simulink model "Feuchtesimulation_G21_EU6AGA_rueckgabewerte"  (R2021b)
settings: Solver=FixedStepAuto  StartTime=start_time  StopTime=stop_time  FixedStep=ts  RelTol=1e-3
undefined symbols (not defined in the file or in its folder): A_Kat0, A_Kat1, A_Kat2, A_Kat3, A_Mantel_Kat0, A_Mantel_Kat1, A_Mantel_Kat2, A_Mantel_Kat3, Air_N2, Air_O2, beladungskennfeld, C_mw, CO2_mw, FeuchteAnsaugluft_rel, FeuchtegradAnsaugluft, Fuel_C, Fuel_H, H2O_mw, H_mw, Kat0_Anzahl_Zonen, Kat1_Anzahl_Zonen, Kat2_Anzahl_Zonen, Kat3_Anzahl_Zonen, l_Kat0, l_Kat1, l_Kat2, l_Kat3, m_Canning_Kat0, m_Canning_Kat1, m_Canning_Kat2, m_Canning_Kat3, m_h2o_kat0_ads, m_h2o_kat0_kond, m_h2o_kat1_ads, m_h2o_kat1_kond, m_h2o_kat2_ads, m_h2o_kat2_kond, m_h2o_kat3_ads, m_h2o_kat3_kond, m_Isolierung_Kat0, m_Isolierung_Kat1, m_Isolierung_Kat2, m_Isolierung_Kat3, m_zeolith_kat0_zone, m_zeolith_kat1_zone, m_zeolith_kat2_zone, m_zeolith_kat3_zone, m_zKat0, m_zKat1, m_zKat2, m_zKat3, Mat_Kat0, Mat_Kat1, Mat_Kat2, Mat_Kat3, N2_mw, O2_mw, p_dsat, Rohr0, Rohr1 ... (+20)
libraries: Feuchtesimulation_Lib x69
(part 1 of 3)
settings Model: SimulationMode=rapid-accelerator  NumberOfSteps=2  SnapshotInterval=1  Creator=QXS2633  LastModifiedBy=q552088
settings SolverCC: AlgebraicLoopSolver=TrustRegion
settings DataIOCC: Decimation=ScopeDecim  SaveOutput=off  SignalLogging=off  DSMLogging=off  SaveTime=off  ReturnWorkspaceOutputs=off
settings DebuggingCC: SFMachineParentedDataDiag=warning  ArithmeticOperatorsInVariantConditions=warning
settings SFSimCC: CustomCodeUndefinedFunction=UseInterfaceOnly

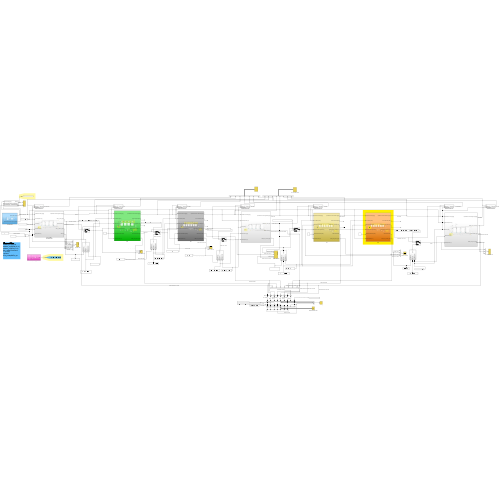
[thumbnail: Simulink's stored preview of the top-level diagram]
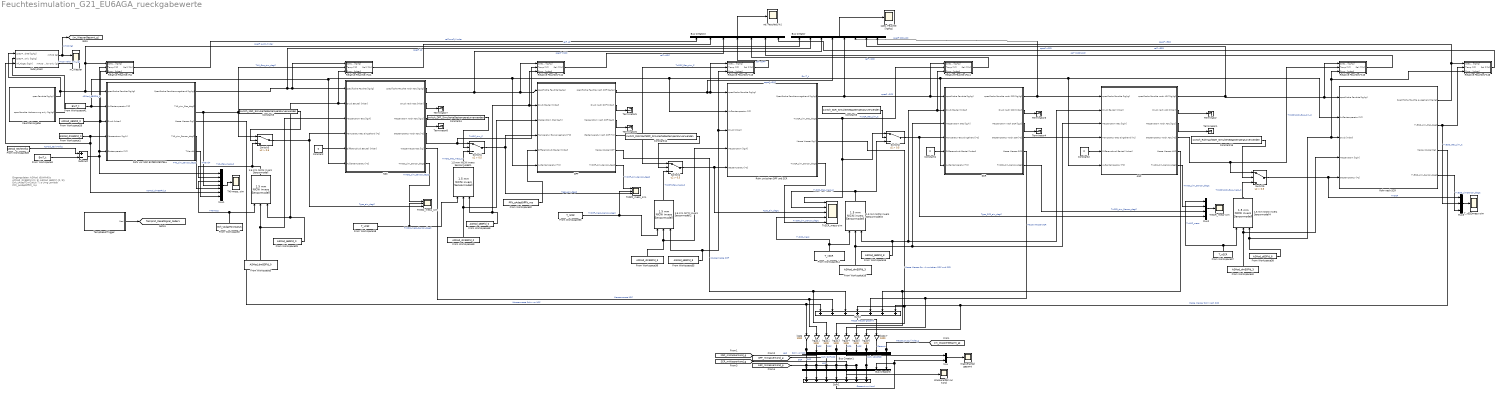
== system Feuchtesimulation_G21_EU6AGA_rueckgabewerte ==
  note: Eingangsdaten:
      | ASMod_tExhMnfUs
      | ASMod_dmEGFld {0 / 3}
      | ASMod_pEGFld {0 / 8}
      | Exh_tAdapTOxiCatUs
      | T / p Umg
      | Lambda
      | PFlt_pAdapDiffFlt_mp
  1.5 mm NiCNi invers Sensormodell{,1..4} (5 alike) : Feuchtesimulation_Lib/1.5 mm NiCNi invers Sensormodell  SystemSampleTime=-1  VariantActivationTime=update diagram  Latency=0  AutoFrameSizeCalculation=off
  ASC : Subsystem
  Bus Creator : BusCreator  Inputs=8
  Bus Creator1 : BusCreator  Inputs=9
  Bus Creator2 : BusCreator  Inputs=7
  Bus Creator3 : BusCreator  Inputs=9
  Constant : Constant  Value=0
  Constant1 : Constant  Value=0
  Constant14 : Constant  Value=switch_RohrNachDPF_SimulierteGastemperaturverwenden
  Constant15 : Constant  Value=switch_RohrnachSCR_SimulierteGastemperaturverwenden
  Constant2 : Constant  Value=0
  Constant3 : Constant  Value=switch_NSC_SimulierteGastemperaturverwenden
  Constant4 : Constant  Value=switch_DPF_SimulierteGastemperaturverwenden
  Constant5 : Constant  Value=switch_SCR_SimulierteGastemperaturverwenden
  DPF : Subsystem
  FeuchteVorgabe : Subsystem
  From Workspace1 : FromWorkspace  VariableName=ASMod_dmEGFld_0  OutputAfterFinalValue=Holding final value
  From Workspace14 : FromWorkspace  VariableName=T_vSCR  OutputAfterFinalValue=Holding final value
  From Workspace15 : FromWorkspace  VariableName=ASMod_pEGFld_8  OutputAfterFinalValue=Holding final value
  From Workspace16 : FromWorkspace  VariableName=ASMod_dmEGFld_3  OutputAfterFinalValue=Holding final value
  From Workspace18 : FromWorkspace  VariableName=T_vCSF  OutputAfterFinalValue=Holding final value
  From Workspace2 : FromWorkspace  VariableName=Exh_tAdapTOxiCatUs  OutputAfterFinalValue=Holding final value
  From Workspace26 : FromWorkspace  VariableName=ASMod_pEGFld_0  OutputAfterFinalValue=Holding final value
  From Workspace28 : FromWorkspace  VariableName=ASMod_tExhMnfUs  OutputAfterFinalValue=Holding final value
  From Workspace29 : FromWorkspace  VariableName=ASMod_pEGFld_0  OutputAfterFinalValue=Holding final value
  From Workspace3 : FromWorkspace  VariableName=EnvT_t
  From Workspace32 : FromWorkspace  VariableName=PFlt_pAdapDiffFlt_mp  OutputAfterFinalValue=Holding final value
  From Workspace33 : FromWorkspace  VariableName=T_nCSF  OutputAfterFinalValue=Holding final value
  From Workspace35 : FromWorkspace  VariableName=ASMod_pEGFld_8  OutputAfterFinalValue=Holding final value
  From Workspace36 : FromWorkspace  VariableName=ASMod_dmEGFld_3  OutputAfterFinalValue=Holding final value
  From Workspace37 : FromWorkspace  VariableName=T_nSCR  OutputAfterFinalValue=Holding final value
  From Workspace38 : FromWorkspace  VariableName=ASMod_pEGFld_8  OutputAfterFinalValue=Holding final value
  From Workspace40 : FromWorkspace  VariableName=ASMod_dmEGFld_3  OutputAfterFinalValue=Holding final value
  From Workspace41 : FromWorkspace  VariableName=EnvT_t  OutputAfterFinalValue=Holding final value
  From Workspace48 : FromWorkspace  VariableName=ASMod_pEGFld_0  OutputAfterFinalValue=Holding final value
  From Workspace49 : FromWorkspace  VariableName=ASMod_dmEGFld_0  OutputAfterFinalValue=Holding final value
  From Workspace5 : FromWorkspace  VariableName=ASMod_dmEGFld_0  OutputAfterFinalValue=Holding final value
  Mux : Mux  Inputs=2
  Mux1 : Mux  Inputs=7
  Mux2 : Mux
  Mux3 : Mux  Inputs=3
  NSC : Subsystem
  Relative Feuchte [%] : Subsystem
  Relative Feuchte [%]1 : Subsystem
  Relative Feuchte [%]2 : Subsystem
  Relative Feuchte [%]3 : Subsystem
  Relative Feuchte [%]4 : Subsystem
  Relative Feuchte [%]5 : Subsystem
  Relative Feuchte [%]6 : Subsystem
  Rohr nach SCR : Subsystem
  Rohr vor NSC EXPERIMENTELL : Subsystem
  Rohr zwischen DPF und SCR : Subsystem
  SCR : Subsystem
  Subsystem : Subsystem
  Subtract : Sum  Inputs=+-
  Sum1 : Sum  Inputs=+++++++
  Sum2 : Sum  Inputs=+++++++
  Switch{1..5} (5 alike) : Switch  Criteria=u2 > Threshold  Threshold=0.5  RndMeth=Simplest  SaturateOnIntegerOverflow=on  InputSameDT=on
  "T40 mess, sim" : Scope
  T_vESDmess-sim : Scope
  TempResetTrigger : Subsystem
  Terminator{,1,3..8} (8 alike) : Terminator
  TnDPF_mess_sim : Scope  NumInputPorts=3
  TnNSC_mess_sim : Scope  NumInputPorts=3
  TnSCR_mess-sim : Scope
  TvSCR_mess-sim : Scope  NumInputPorts=5
  Wasseranfall gesamt : Scope
  Wasseranfall nur Kond : Scope
  kg2g {,1..7} (8 alike) : Gain  Gain=1000
  m_Wasser : Scope  NumInputPorts=2
  rel. Feuchte [%] : Scope
  spez. Feuchte [kg/kg] : Scope
  tag scope: TempInit_ResetSignal_0oder1=global
  wires:
  Sum2/1 -> kg2g 7/1  "Masse Wasser gesamt"
  NSC/3(Massenstrom nach NSC [kg/s]) -> Terminator8/1
  [SCR_mWasserKond_g] -> Sum1/5, Bus Creator3/5  "SCR"
  Constant2/1 -> ASC/5(Differenzdruck Bauteil [mbar])
  Bus Creator3/1 -> Wasseranfall nur Kond/1
  Relative Feuchte [%]2/1(Rel F [%]) -> Bus Creator2/3  "relF nNSC"
  Sum1/1 -> Mux/2, Bus Creator3/8  "Gesamt nur Kond"
  kg2g 4/1 -> Bus Creator1/5  "SCR"
  Constant5/1 -> Switch2/2
  Rohr zwischen DPF und SCR/3(Masse Wasser [kg]) -> kg2g 3/1, Sum2/4  "Masse Wasser Rorh zwischen DPF und SCR"
  SCR/1(spezifische Feuchte nach SCR [kg/kg]) -> ASC/1(spezifische Feuchte [kg/kg]), Bus Creator/6  "spezF SCR-ASC"
  Rohr nach SCR/3(Masse Wasser [kg]) -> Sum2/7, kg2g 6/1  "Masse Wasser Rohr nach SCR"
  Switch5/1 -> Rohr nach SCR/5(Gastemperatur [°C]), Mux3/1  "TnSCR"
  [m_WasserGesamt_g] -> Bus Creator3/9, Bus Creator1/9  "Wasser_ausZylinder_g"
  ASC/3(Massenstrom nach ASC [kg/s]) -> Terminator1/1
  SCR/2(Druck nach SCR [mbar]) -> Terminator3/1
  ASC/2(Druck nach ASC [mbar]) -> Terminator/1
  kg2g 3/1 -> Sum1/4, Bus Creator3/4, Bus Creator1/4  "Rohr DPF-SCR"
  Relative Feuchte [%]4/1(Rel F [%]) -> Bus Creator2/5  "relF vSCR"
  [NSC_mWasserKond_g] -> Sum1/2, Bus Creator3/2  "NSC"
  Subsystem/1(mH2O [g]) -> m_Wasser/1, [m_WasserGesamt_g]  "mH2O [g]"
  kg2g 6/1 -> Sum1/7, Bus Creator3/7, Bus Creator1/7  "Rohr ASC-ESD"
  "kg2g "/1 -> Sum1/1, Bus Creator3/1, Bus Creator1/1  "Rohr vor NSC"
  Relative Feuchte [%]/1(Rel F [%]) -> Bus Creator2/1  "relF ausZylinder"
  Bus Creator1/1 -> Mux/1
  SCR/3(Massenstrom nach SCR [kg/s]) -> Terminator4/1
  Relative Feuchte [%]3/1(Rel F [%]) -> Bus Creator2/4  "relF nDPF"
  FeuchteVorgabe/2(spez.Feuchte Verbrennung only [kg/kg]) -> Subsystem/2(spez-Feuchte Verbrennung only [kg/kg])
  DPF/3(Massenstrom nach DPF [kg/s]) -> Terminator6/1
  Rohr nach SCR/1(Spezifische Feuchte ausgehend [kg/kg]) -> Relative Feuchte [%]6/1(Spez F [kg/kg]), Bus Creator/8  "spezF vESD"
  DPF/4(Gastemperatur nach DPF [°C]) -> Switch4/1, Relative Feuchte [%]3/2(Temp [°C])  "TnDPF_Gas_sim_C"
  Constant15/1 -> Switch5/2
  [DPF_mWasserKond_g] -> Sum1/3, Bus Creator3/3  "DPF"
  kg2g 5/1 -> Bus Creator1/6  "ASC"
  ASC/4(Gastemperatur nach ASC [°C]) -> Relative Feuchte [%]5/2(Temp [°C]), Switch5/1  "TnSCR(ASC)_Gas_sim_C"
  FeuchteVorgabe/1(spez.Feuchte [kg/kg]) -> Subsystem/1(spez-Feuchte [kg/kg]), Bus Creator/1, Relative Feuchte [%]/1(Spez F [kg/kg]), Rohr vor NSC EXPERIMENTELL/1(spezifische Feuchte [kg/kg])  "spezF ausZylinder"
  Switch3/1 -> TnNSC_mess_sim/3, NSC/4(Temperatur Gas eingehend [°C])  "Tgas_ein_degC"
  ASC/5(Masse Wasser ASC) -> Sum2/6, kg2g 5/1
  kg2g 7/1 -> Bus Creator1/8  "Gesamt"
  From Workspace18/1 -> TnNSC_mess_sim/2, 1.5 mm NiCNi invers Sensormodell1/1  "TnNSC_mess_Sensor_degC"
  Rohr vor NSC EXPERIMENTELL/2(T40_sim_Gas_degC) -> Mux1/4, Switch3/1, Relative Feuchte [%]1/2(Temp [°C])  "T40_Gas_sim_degC"
  1.5 mm NiCNi invers Sensormodell2/1 -> Switch4/3  "TnDPF_Gas_mess_C"
  1.5 mm NiCNi invers Sensormodell4/1 -> Switch5/3  "TnSCR(ASC)_Gas_mess_C"
  Switch4/1 -> TvSCR_mess-sim/3, Rohr zwischen DPF und SCR/5(Gastemperatur [°C])  "Tgas_ein_degC"
  Rohr zwischen DPF und SCR/2(TvSCR_sim_Gas_degC) -> Relative Feuchte [%]4/2(Temp [°C]), TvSCR_mess-sim/1, Switch2/1  "TvSCR_Gas_sim_C"
  NSC/2(Druck nach NSC [mbar]) -> Terminator7/1
  Relative Feuchte [%]5/1(Rel F [%]) -> Bus Creator2/6  "relF nSCR(ASC)"
  Rohr nach SCR/2(TvESD_sim_Gas_degC) -> Relative Feuchte [%]6/2(Temp [°C]), Mux3/2  "TvESD_Gas_sim_C"
  DPF/2(Druck nach DPF [mbar]) -> Terminator5/1
  Rohr vor NSC EXPERIMENTELL/3(Masse Wasser [kg]) -> "kg2g "/1, Sum2/1  "Wassermasse Rohr vor NSC"
  Rohr vor NSC EXPERIMENTELL/1(Spezifische Feuchte ausgehend [kg/kg]) -> Bus Creator/2, Relative Feuchte [%]1/1(Spez F [kg/kg]), NSC/1(spezifische Feuchte [kg/kg])  "spezF 40"
  Switch2/1 -> Mux2/4, SCR/4(Temperatur Gas eingehend [°C])  "Tgas_SCR_ein_degC"
  [ASC_mWasserKond_g] -> Sum1/6, Bus Creator3/6  "ASC"
  From Workspace41/1 -> NSC/6(Außentemperatur [°C]), SCR/6(Außentemperatur [°C]), Rohr nach SCR/2(Außentemperatur [°C]), ASC/6(Außentemperatur [°C]), Rohr zwischen DPF und SCR/2(Außentemperatur [°C]), DPF/6(Außentemperatur [°C]), Rohr vor NSC EXPERIMENTELL/2(Außentemperatur [°C])  "EnvT_t"
  From Workspace28/1 -> Subtract/1  "ASMod_tExhMnfUs"
  Rohr zwischen DPF und SCR/1(Spezifische Feuchte ausgehend [kg/kg]) -> Relative Feuchte [%]4/1(Spez F [kg/kg]), SCR/1(spezifische Feuchte [kg/kg]), Bus Creator/5  "spezF vSCR"
  Bus Creator2/1 -> rel. Feuchte [%]/1
  From Workspace1/1 -> Mux1/6, Subsystem/3(mf_Abgas [kg/h]), Rohr vor NSC EXPERIMENTELL/4(Massenstrom [kg/h])  "ASMod_dmEGFld_0"
  From Workspace37/1 -> Mux2/1, 1.5 mm NiCNi invers Sensormodell4/1  "TnASC_mess"
  From Workspace26/1 -> Relative Feuchte [%]/3(Druck [mbar]), Rohr vor NSC EXPERIMENTELL/3(Druck [mbar])  "ASMod_pEGFld_0"
  From Workspace29/1 -> Relative Feuchte [%]1/3(Druck [mbar]), NSC/2(Druck Bauteil [mbar]), 1.5 mm NiCNi invers Sensormodell/3
  Subsystem/2(mH2O Verbr.-only [g]) -> m_Wasser/2  "mH2O Verbr. only [g]"
  Mux/1 -> Wasseranfall gesamt/1
  ASC/1(spezifische Feuchte nach ASC [kg/kg]) -> Relative Feuchte [%]5/1(Spez F [kg/kg]), Rohr nach SCR/1(spezifische Feuchte [kg/kg]), Bus Creator/7  "spezF nSCR"
  From Workspace33/1 -> TnDPF_mess_sim/2, 1.5 mm NiCNi invers Sensormodell2/1  "TnDPF_mess_Sensor_degC"
  DPF/1(spezifische Feuchte nach DPF [kg/kg]) -> Rohr zwischen DPF und SCR/1(spezifische Feuchte [kg/kg]), Relative Feuchte [%]3/1(Spez F [kg/kg]), Bus Creator/4  "spezF nDPF"
  Relative Feuchte [%]1/1(Rel F [%]) -> Bus Creator2/2  "relF 40"
  NSC/1(spezifische Feuchte nach NSC [kg/kg]) -> Bus Creator/3, Relative Feuchte [%]2/1(Spez F [kg/kg]), DPF/1(spezifische Feuchte [kg/kg])  "spezF nNSC"
  DPF/5(Masse Wasser DPF) -> kg2g 2/1, Sum2/3  "Wassermasse DPF"
  From Workspace38/1 -> Relative Feuchte [%]6/3(Druck [mbar]), Relative Feuchte [%]5/3(Druck [mbar]), Rohr nach SCR/3(Druck [mbar]), 1.5 mm NiCNi invers Sensormodell4/3
  From Workspace2/1 -> Mux1/3, 1.5 mm NiCNi invers Sensormodell/1  "T40mess"
  1.5 mm NiCNi invers Sensormodell/1 -> Mux1/2, Switch3/3  "T40_Gas_mess_C"
  NSC/5(Wassermasse NSC [kg]) -> kg2g 1/1, Sum2/2  "Wassermasse NSC"
  Constant4/1 -> Switch1/2
  kg2g 2/1 -> Bus Creator1/3  "DPF"
  Constant3/1 -> Switch3/2
  From Workspace15/1 -> ASC/2(Druck Bauteil [mbar]), Relative Feuchte [%]4/3(Druck [mbar]), SCR/2(Druck Bauteil [mbar]), 1.5 mm NiCNi invers Sensormodell3/3
  From Workspace40/1 -> Rohr nach SCR/4(Massenstrom [kg/h]), 1.5 mm NiCNi invers Sensormodell4/2
  NSC/6(TnNSC_sim_Sensor_degC) -> TnNSC_mess_sim/1  "TnNSC_sim_Sensor_degC"
  Constant14/1 -> Switch4/2
  From Workspace36/1 -> Rohr zwischen DPF und SCR/4(Massenstrom [kg/h]), 1.5 mm NiCNi invers Sensormodell2/2
  From Workspace48/1 -> DPF/2(Druck Bauteil [mbar]), Relative Feuchte [%]2/3(Druck [mbar]), 1.5 mm NiCNi invers Sensormodell1/3
  From Workspace35/1 -> Relative Feuchte [%]3/3(Druck [mbar]), Rohr zwischen DPF und SCR/3(Druck [mbar]), 1.5 mm NiCNi invers Sensormodell2/3
  1.5 mm NiCNi invers Sensormodell1/1 -> Switch1/3  "TnNSC_Gas_mess_C"
  Bus Creator/1 -> spez. Feuchte [kg/kg]/1
  NSC/4(Gastemperatur nach NSC [°C]) -> Relative Feuchte [%]2/2(Temp [°C]), Switch1/1  "TnNSC_sim_C"
  From Workspace32/1 -> DPF/5(Differenzdruck Bauteil [mbar])
  SCR/4(Gastemperatur nach SCR [°C]) -> ASC/4(Temperatur Gas eingehend [°C])
  kg2g 1/1 -> Bus Creator1/2  "NSC"
  From Workspace49/1 -> DPF/3(Massenstrom Gas [kg/h]), 1.5 mm NiCNi invers Sensormodell1/2
  From Workspace14/1 -> TvSCR_mess-sim/4, 1.5 mm NiCNi invers Sensormodell3/1  "TvSCR_mess"
  1.5 mm NiCNi invers Sensormodell3/1 -> TvSCR_mess-sim/2, Switch2/3  "TvSCR_Gas_mess_C"
  SCR/5(Masse Wasser SCR) -> Sum2/5, kg2g 4/1  "Masse Wasser SCR"
  Switch1/1 -> TnDPF_mess_sim/3, DPF/4(Temperatur Gas eingehend [°C])  "Tgas_ein_degC"
  ASC/6(TnASC_sim_Sensor_degC) -> Mux2/2  "TnASC_sim_Sensor_degC"
  Constant1/1 -> SCR/5(Differenzdruck Bauteil [mbar])
  From Workspace16/1 -> ASC/3(Massenstrom Gas [kg/h]), SCR/3(Massenstrom Gas [kg/h]), 1.5 mm NiCNi invers Sensormodell3/2
  Constant/1 -> NSC/5(Differenzdruck Bauteil [mbar])
  From Workspace5/1 -> NSC/3(Massenstrom Gas [kg/h]), 1.5 mm NiCNi invers Sensormodell/2
  TempResetTrigger/1(Resi) -> [TempInit_ResetSignal_0oder1]
  Mux1/1 -> "T40 mess, sim"/1
  Rohr vor NSC EXPERIMENTELL/4(T40_sim_Sensor_degC) -> Mux1/5  "T40_sim_Sensor_degC"
  DPF/6(TnDPF_sim_Sensor_degC) -> TnDPF_mess_sim/1  "TnDPF_sim_Sensor_degC"
  Rohr zwischen DPF und SCR/4(TvSCR_sim_Sensor_degC) -> TvSCR_mess-sim/5  "TvSCR_sim_Sensor_degC"
  Mux2/1 -> TnSCR_mess-sim/1
  SCR/6(TnSCR_sim_Sensor_degC) -> Mux2/3  "TnSCR_sim_Sensor_degC"
  Mux3/1 -> T_vESDmess-sim/1
  Rohr nach SCR/4(TvESD_sim_Sensor_degC) -> Mux3/3  "TvESD_simSensor_degC"
  Rohr vor NSC EXPERIMENTELL/5(TWand4) -> Mux1/7  "TWand4"
  Relative Feuchte [%]6/1(Rel F [%]) -> Bus Creator2/7  "relF vESD"
  Subtract/1 -> Rohr vor NSC EXPERIMENTELL/5(Gastemperatur [°C]), Relative Feuchte [%]/2(Temp [°C]), Mux1/1
  From Workspace3/1 -> Subtract/2

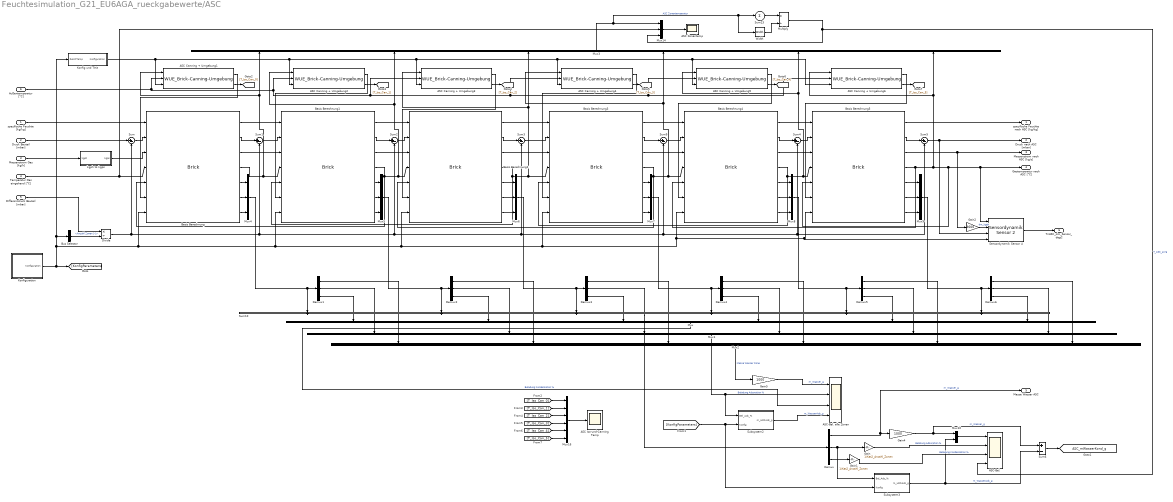
== system Feuchtesimulation_G21_EU6AGA_rueckgabewerte/ASC ==
  spezifische Feuchte [kg/kg] : Inport
  Druck Bauteil [mbar] : Inport  Port=2
  Massenstrom Gas [kg/h] : Inport  Port=3
  Temperatur Gas eingehend [°C] : Inport  Port=4
  Differenzdruck Bauteil [mbar] : Inport  Port=5
  Außentemperatur [°C] : Inport  Port=6
  ASC Canning + Umgebung{1..6} (6 alike) : Feuchtesimulation_Lib/WUE_Brick-Canning-Umgebung  SystemSampleTime=-1  VariantActivationTime=update diagram  Latency=0  AutoFrameSizeCalculation=off
  ASC Iso-und-CanningTemp : Scope
  ASC Zonentemp : Scope
  ASC-Bel. : Scope  NumInputPorts=4
  ASC-Bel. alle Zonen : Scope  NumInputPorts=4
  Basis Berechnung{,1..5} (6 alike) : Feuchtesimulation_Lib/Brick  SystemSampleTime=-1  VariantActivationTime=update diagram  Latency=0  AutoFrameSizeCalculation=off
  Bus Selector : BusSelector  OutputSignals=Anzahl Zonen [-]
  Demux{,1..6} (7 alike) : Demux  Outputs=3
  Divide : Product  Inputs=*/
  Gain : Gain  Gain=1/Kat2_Anzahl_Zonen
  Gain1 : Gain  Gain=1/Kat2_Anzahl_Zonen
  Gain2 : Gain  Gain=3600
  Gain4 : Gain  Gain=1000
  Gain5 : Gain  Gain=1000
  Konfig und TInit : Subsystem
  Konfiguration : Subsystem
  Multiply : Product  Inputs=*/
  Mux{,1..3,16} (5 alike) : Mux  Inputs=6
  Mux10 : Mux  Inputs=2
  Mux{4..9,14} (7 alike) : Mux  Inputs=3
  Sensordynamik Sensor 4 : Feuchtesimulation_Lib/Sensordynamik Sensor 2  SystemSampleTime=-1  VariantActivationTime=update diagram  Latency=0  AutoFrameSizeCalculation=off
  Subsystem2 : Subsystem
  Subsystem3 : Subsystem
  Sum{,1..5,9} (7 alike) : Sum  Inputs=|+-
  Sum10 : Sum  Inputs=++++++
  Sum13 : Sum  Inputs=+
  Sum6 : Sum  Inputs=+-
  Width : Width
  kgph to kgps : Subsystem
  spezifische Feuchte nach ASC [kg/kg] : Outport  VectorParamsAs1DForOutWhenUnconnected=off
  Druck nach ASC [mbar] : Outport  Port=2  VectorParamsAs1DForOutWhenUnconnected=off
  Massenstrom nach ASC [kg/s] : Outport  Port=3  VectorParamsAs1DForOutWhenUnconnected=off
  Gastemperatur nach ASC [°C] : Outport  Port=4  VectorParamsAs1DForOutWhenUnconnected=off
  Masse Wasser ASC : Outport  Port=5  VectorParamsAs1DForOutWhenUnconnected=off
  TnASC_sim_Sensor_degC : Outport  Port=6  VectorParamsAs1DForOutWhenUnconnected=off
  tag scope: ASC_mWasserKond_g=global
  wires:
  Demux2/2 -> Mux1/2
  Basis Berechnung3/4 -> Basis Berechnung4/4, ASC Canning + Umgebung4/1, Mux3/4, Basis Berechnung2/5
  Basis Berechnung2/4 -> Basis Berechnung1/5, Basis Berechnung3/4, ASC Canning + Umgebung3/1, Mux3/3
  Basis Berechnung4/4 -> Basis Berechnung3/5, Basis Berechnung5/4, Mux3/5, ASC Canning + Umgebung5/1
  Sum9/1 -> Basis Berechnung4/2
  Basis Berechnung5/1 -> spezifische Feuchte nach ASC [kg/kg]/1
  Basis Berechnung/5 -> Mux4/1
  Basis Berechnung3/3 -> Basis Berechnung4/3
  Basis Berechnung/3 -> Basis Berechnung1/3
  Basis Berechnung5/6 -> Mux9/2
  Sum4/1 -> Basis Berechnung5/2
  Basis Berechnung1/4 -> Basis Berechnung/5, Basis Berechnung2/4, ASC Canning + Umgebung2/1, Mux3/2
  Basis Berechnung2/3 -> Basis Berechnung3/3
  Basis Berechnung1/3 -> Basis Berechnung2/3
  Sum3/1 -> Basis Berechnung3/2
  Basis Berechnung2/6 -> Mux6/2
  Basis Berechnung4/6 -> Mux8/2
  Bus Selector/1 -> Divide/2  "<Anzahl Zonen [-]>"
  Basis Berechnung/7 -> Mux4/3
  Divide/1 -> Sum5/2, Sum4/2, Sum9/2, Sum3/2, Sum2/2, Sum1/2, Sum/2
  Basis Berechnung3/1 -> Basis Berechnung4/1
  Basis Berechnung1/5 -> Mux5/1
  Basis Berechnung1/6 -> Mux5/2
  Basis Berechnung1/7 -> Mux5/3
  Massenstrom Gas [kg/h]/1 -> kgph to kgps/1(kgph)
  Basis Berechnung/6 -> Mux4/2
  Basis Berechnung2/7 -> Mux6/3
  Basis Berechnung4/7 -> Mux8/3
  Basis Berechnung4/3 -> Basis Berechnung5/3
  kgph to kgps/1(kgps) -> Basis Berechnung/3
  Basis Berechnung5/7 -> Mux9/3
  Sum2/1 -> Basis Berechnung2/2
  Basis Berechnung4/1 -> Basis Berechnung5/1
  Differenzdruck Bauteil [mbar]/1 -> Divide/1
  spezifische Feuchte [kg/kg]/1 -> Basis Berechnung/1
  Basis Berechnung2/5 -> Mux6/1
  Demux5/2 -> Mux1/5
  Basis Berechnung/1 -> Basis Berechnung1/1
  Basis Berechnung/4 -> Basis Berechnung1/4, ASC Canning + Umgebung1/1, Mux3/1
  Demux6/1 -> Mux2/6
  Basis Berechnung4/2 -> Sum4/1
  Demux6/2 -> Mux1/6
  Druck Bauteil [mbar]/1 -> Sum/1
  Demux5/1 -> Mux2/5
  Basis Berechnung1/1 -> Basis Berechnung2/1
  Demux6/3 -> Mux/6
  Basis Berechnung2/1 -> Basis Berechnung3/1
  Basis Berechnung5/5 -> Mux9/1
  Demux5/3 -> Mux/5
  Demux2/3 -> Mux/2
  Basis Berechnung3/5 -> Mux7/1
  Demux3/3 -> Mux/3
  Sum1/1 -> Basis Berechnung1/2
  Demux4/1 -> Mux2/4
  Demux1/1 -> Mux2/1
  Demux2/1 -> Mux2/2
  Demux3/1 -> Mux2/3
  Basis Berechnung3/6 -> Mux7/2
  Demux1/3 -> Mux/1
  Basis Berechnung/2 -> Sum1/1
  Basis Berechnung3/2 -> Sum9/1
  Demux4/2 -> Mux1/4
  Sum/1 -> Basis Berechnung/2
  Basis Berechnung1/2 -> Sum2/1
  Basis Berechnung4/5 -> Mux8/1
  Basis Berechnung2/2 -> Sum3/1
  Basis Berechnung5/2 -> Sum5/1
  Demux1/2 -> Mux1/1
  Demux3/2 -> Mux1/3
  Demux4/3 -> Mux/4
  Basis Berechnung3/7 -> Mux7/3
  Außentemperatur [°C]/1 -> ASC Canning + Umgebung1/2, ASC Canning + Umgebung6/2, ASC Canning + Umgebung5/2, ASC Canning + Umgebung4/2, ASC Canning + Umgebung3/2, ASC Canning + Umgebung2/2
  ASC Canning + Umgebung1/1 -> Basis Berechnung/6
  ASC Canning + Umgebung2/1 -> Basis Berechnung1/6
  ASC Canning + Umgebung3/1 -> Basis Berechnung2/6
  ASC Canning + Umgebung4/1 -> Basis Berechnung3/6
  ASC Canning + Umgebung5/1 -> Basis Berechnung4/6
  ASC Canning + Umgebung6/1 -> Basis Berechnung5/6
  Mux4/1 -> Demux1/1, Sum10/1
  Mux5/1 -> Sum10/2, Demux2/1
  Mux6/1 -> Sum10/3, Demux3/1
  Mux7/1 -> Demux4/1, Sum10/4
  Mux8/1 -> Demux5/1, Sum10/5
  Mux9/1 -> Sum10/6, Demux6/1
  Gain4/1 -> Sum6/1, Mux10/1  "m_Wasser_g"
  Demux/3 -> Gain1/1
  Sum10/1 -> Demux/1
  Demux/2 -> Subsystem3/1(Bel_Ads_%), Gain/1
  [KonfigParameters] -> Subsystem2/2(Konfig), Subsystem3/2(Konfig)
  Mux1/1 -> ASC-Bel. alle Zonen/2, Subsystem2/1(Bel_Ads_%)  "Beladung Adsorption %"
  Mux/1 -> ASC-Bel. alle Zonen/3  "Beladung Kondensation %"
  Gain/1 -> ASC-Bel./2  "Belatung Adsorption %"
  Mux2/1 -> Gain5/1  "Masse Wasser Zone"
  Gain1/1 -> ASC-Bel./3  "Beladung Kondensation %"
  Subsystem3/1(m_H2OAds_g) -> Sum6/2, Mux10/2  "m_WasserAds_g"
  Subsystem2/1(m_H2OAds_g) -> ASC-Bel. alle Zonen/4  "m_WasserAds_g"
  Mux10/1 -> ASC-Bel./1
  Gain5/1 -> ASC-Bel. alle Zonen/1  "m_Wasser_g"
  Demux/1 -> Masse Wasser ASC/1, Gain4/1  "m_Wasser_g"
  Sum6/1 -> [ASC_mWasserKond_g]
  Width/1 -> Multiply/2
  Multiply/1 -> ASC-Bel./4, Mux14/3  "T_ASC_avrg"
  Mux14/1 -> ASC Zonentemp/1
  Temperatur Gas eingehend [°C]/1 -> Mux14/2, Basis Berechnung/4
  Sum13/1 -> Multiply/1
  Mux3/1 -> Sum13/1, Width/1, Mux14/1  "ASC Zonentemperatur"
  Konfig und TInit/1(Konfiguration) -> ASC Canning + Umgebung1/3, ASC Canning + Umgebung2/3, ASC Canning + Umgebung3/3, ASC Canning + Umgebung4/3, ASC Canning + Umgebung5/3, ASC Canning + Umgebung6/3
  [T_Iso_Can_3] -> Mux16/4
  [T_Iso_Can_2] -> Mux16/3
  [T_Iso_Can_0] -> Mux16/1
  [T_Iso_Can_5] -> Mux16/6
  [T_Iso_Can_4] -> Mux16/5
  [T_Iso_Can_1] -> Mux16/2
  Mux16/1 -> ASC Iso-und-CanningTemp/1
  ASC Canning + Umgebung1/2 -> [T_Iso_Can_0]
  ASC Canning + Umgebung2/2 -> [T_Iso_Can_1]
  ASC Canning + Umgebung3/2 -> [T_Iso_Can_2]
  ASC Canning + Umgebung4/2 -> [T_Iso_Can_3]
  ASC Canning + Umgebung5/2 -> [T_Iso_Can_4]
  ASC Canning + Umgebung6/2 -> [T_Iso_Can_5]
  Sum5/1 -> Sensordynamik Sensor 4/3, Druck nach ASC [mbar]/1
  Basis Berechnung5/3 -> Gain2/1, Massenstrom nach ASC [kg/s]/1
  Gain2/1 -> Sensordynamik Sensor 4/2  "dm_kgph"
  Sensordynamik Sensor 4/1 -> TnASC_sim_Sensor_degC/1
  Basis Berechnung5/4 -> Basis Berechnung4/5, Basis Berechnung5/5, Sensordynamik Sensor 4/1, Gastemperatur nach ASC [°C]/1, Mux3/6, ASC Canning + Umgebung6/1
  Konfiguration/1(Konfiguration) -> [KonfigParameters], Sensordynamik Sensor 4/4, Basis Berechnung5/7, Basis Berechnung4/7, Basis Berechnung3/7, Basis Berechnung2/7, Basis Berechnung1/7, Basis Berechnung/7, Konfig und TInit/1(ReInitTemp), Bus Selector/1

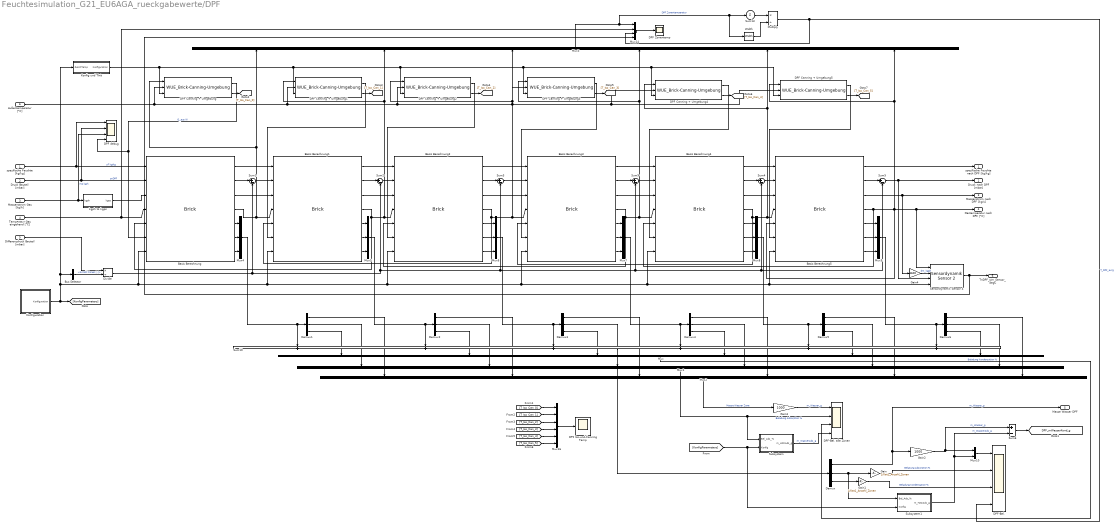
== system Feuchtesimulation_G21_EU6AGA_rueckgabewerte/DPF ==
  spezifische Feuchte [kg/kg] : Inport
  Druck Bauteil [mbar] : Inport  Port=2
  Massenstrom Gas [kg/h] : Inport  Port=3
  Temperatur Gas eingehend [°C] : Inport  Port=4
  Differenzdruck Bauteil [mbar] : Inport  Port=5
  Außentemperatur [°C] : Inport  Port=6
  Basis Berechnung{,1..5} (6 alike) : Feuchtesimulation_Lib/Brick  SystemSampleTime=-1  VariantActivationTime=update diagram  Latency=0  AutoFrameSizeCalculation=off
  Bus Selector : BusSelector  OutputSignals=Anzahl Zonen [-]
  DPF Canning + Umgebung{,1..5} (6 alike) : Feuchtesimulation_Lib/WUE_Brick-Canning-Umgebung  SystemSampleTime=-1  VariantActivationTime=update diagram  Latency=0  AutoFrameSizeCalculation=off
  DPF Iso-und-CanningTemp : Scope
  DPF Zonentemp : Scope
  DPF debug : Scope  NumInputPorts=4
  DPF-Bel. : Scope  NumInputPorts=4
  DPF-Bel. alle Zonen : Scope  NumInputPorts=4
  Demux{,1..6} (7 alike) : Demux  Outputs=3
  Divide : Product  Inputs=*/
  Gain : Gain  Gain=1/Kat1_Anzahl_Zonen
  Gain1 : Gain  Gain=1/Kat1_Anzahl_Zonen
  Gain2 : Gain  Gain=1000
  Gain3 : Gain  Gain=1000
  Gain4 : Gain  Gain=3600
  Konfig und TInit : Subsystem
  Konfiguration : Subsystem
  Multiply : Product  Inputs=*/
  Mux{,1..3,16} (5 alike) : Mux  Inputs=6
  Mux10 : Mux  Inputs=2
  Mux14 : Mux
  Mux{4..9} (6 alike) : Mux  Inputs=3
  Sensordynamik Sensor 4 : Feuchtesimulation_Lib/Sensordynamik Sensor 2  SystemSampleTime=-1  VariantActivationTime=update diagram  Latency=0  AutoFrameSizeCalculation=off
  Subsystem : Subsystem
  Subsystem1 : Subsystem
  Sum{1..5,9} (6 alike) : Sum  Inputs=|+-
  Sum10 : Sum  Inputs=++++++
  Sum13 : Sum  Inputs=+
  Sum6 : Sum  Inputs=+-
  Width : Width
  kgph to kgps : Subsystem
  spezifische Feuchte nach DPF [kg/kg] : Outport  VectorParamsAs1DForOutWhenUnconnected=off
  Druck nach DPF [mbar] : Outport  Port=2  VectorParamsAs1DForOutWhenUnconnected=off
  Massenstrom nach DPF [kg/s] : Outport  Port=3  VectorParamsAs1DForOutWhenUnconnected=off
  Gastemperatur nach DPF [°C] : Outport  Port=4  VectorParamsAs1DForOutWhenUnconnected=off
  Masse Wasser DPF : Outport  Port=5  VectorParamsAs1DForOutWhenUnconnected=off
  TnDPF_sim_Sensor_degC : Outport  Port=6  VectorParamsAs1DForOutWhenUnconnected=off
  tag scope: DPF_mWasserKond_g=global
  wires:
  Demux2/2 -> Mux1/2
  Basis Berechnung3/4 -> Basis Berechnung4/4, DPF Canning + Umgebung3/1, Mux3/4, Basis Berechnung2/5
  Basis Berechnung2/4 -> Basis Berechnung1/5, Basis Berechnung3/4, DPF Canning + Umgebung2/1, Mux3/3
  Basis Berechnung4/4 -> Basis Berechnung3/5, Basis Berechnung5/4, Mux3/5, DPF Canning + Umgebung4/1
  Sum9/1 -> Basis Berechnung4/2
  Basis Berechnung5/1 -> spezifische Feuchte nach DPF [kg/kg]/1
  Basis Berechnung/5 -> Mux4/1
  Basis Berechnung3/3 -> Basis Berechnung4/3
  Basis Berechnung/3 -> Basis Berechnung1/3
  Basis Berechnung5/6 -> Mux9/2
  Sum4/1 -> Basis Berechnung5/2
  Basis Berechnung1/4 -> Basis Berechnung/5, Basis Berechnung2/4, DPF Canning + Umgebung1/1, Mux3/2
  Basis Berechnung2/3 -> Basis Berechnung3/3
  Basis Berechnung1/3 -> Basis Berechnung2/3
  Sum3/1 -> Basis Berechnung3/2
  Basis Berechnung2/6 -> Mux6/2
  Basis Berechnung4/6 -> Mux8/2
  Bus Selector/1 -> Divide/2  "<Anzahl Zonen [-]>"
  Basis Berechnung/7 -> Mux4/3
  Divide/1 -> Sum5/2, Sum4/2, Sum9/2, Sum3/2, Sum2/2, Sum1/2
  Basis Berechnung3/1 -> Basis Berechnung4/1
  Basis Berechnung1/5 -> Mux5/1
  Basis Berechnung1/6 -> Mux5/2
  Basis Berechnung1/7 -> Mux5/3
  Massenstrom Gas [kg/h]/1 -> DPF debug/3, kgph to kgps/1(kgph)  "mp kg/h"
  Basis Berechnung/6 -> Mux4/2
  Basis Berechnung2/7 -> Mux6/3
  Basis Berechnung4/7 -> Mux8/3
  Basis Berechnung4/3 -> Basis Berechnung5/3
  kgph to kgps/1(kgps) -> Basis Berechnung/3
  Gain/1 -> DPF-Bel./2  "Belatung Adsorption %"
  Basis Berechnung5/7 -> Mux9/3
  Sum2/1 -> Basis Berechnung2/2
  Demux/3 -> Gain1/1
  Mux2/1 -> Gain3/1  "Masse Wasser Zone"
  Basis Berechnung4/1 -> Basis Berechnung5/1
  Differenzdruck Bauteil [mbar]/1 -> Divide/1
  spezifische Feuchte [kg/kg]/1 -> DPF debug/1, Basis Berechnung/1  "sF kg/kg"
  Basis Berechnung2/5 -> Mux6/1
  Demux5/2 -> Mux1/5
  Mux1/1 -> DPF-Bel. alle Zonen/2, Subsystem/1(Bel_Ads_%)  "Beladung Adsorption %"
  Basis Berechnung/1 -> Basis Berechnung1/1
  Basis Berechnung/4 -> Basis Berechnung1/4, DPF Canning + Umgebung/1, Mux3/1
  Demux6/1 -> Mux2/6
  Basis Berechnung4/2 -> Sum4/1
  Demux6/2 -> Mux1/6
  Demux5/1 -> Mux2/5
  Basis Berechnung1/1 -> Basis Berechnung2/1
  Demux6/3 -> Mux/6
  Gain1/1 -> DPF-Bel./3  "Beladung Kondensation %"
  Temperatur Gas eingehend [°C]/1 -> Mux14/2, Basis Berechnung/4
  Basis Berechnung2/1 -> Basis Berechnung3/1
  Basis Berechnung5/5 -> Mux9/1
  Demux/2 -> Subsystem1/1(Bel_Ads_%), Gain/1
  Demux5/3 -> Mux/5
  Demux/1 -> Masse Wasser DPF/1, Gain2/1  "m_Wasser_g"
  Demux2/3 -> Mux/2
  Basis Berechnung3/5 -> Mux7/1
  Demux3/3 -> Mux/3
  Sum1/1 -> Basis Berechnung1/2
  Sum10/1 -> Demux/1
  Demux4/1 -> Mux2/4
  Demux1/1 -> Mux2/1
  Demux2/1 -> Mux2/2
  Demux3/1 -> Mux2/3
  Basis Berechnung3/6 -> Mux7/2
  Demux1/3 -> Mux/1
  Basis Berechnung/2 -> Sum1/1
  Mux/1 -> DPF-Bel. alle Zonen/3  "Beladung Kondensation %"
  Basis Berechnung3/2 -> Sum9/1
  Demux4/2 -> Mux1/4
  Druck Bauteil [mbar]/1 -> DPF debug/2, Basis Berechnung/2  "pvDPF"
  Basis Berechnung1/2 -> Sum2/1
  Basis Berechnung4/5 -> Mux8/1
  Basis Berechnung2/2 -> Sum3/1
  Basis Berechnung5/2 -> Sum5/1
  Demux1/2 -> Mux1/1
  Demux3/2 -> Mux1/3
  Demux4/3 -> Mux/4
  Basis Berechnung3/7 -> Mux7/3
  Außentemperatur [°C]/1 -> DPF Canning + Umgebung/2, DPF Canning + Umgebung1/2, DPF Canning + Umgebung2/2, DPF Canning + Umgebung3/2, DPF Canning + Umgebung5/2, DPF Canning + Umgebung4/2
  DPF Canning + Umgebung/1 -> DPF debug/4, Basis Berechnung/6  "Q_aus W"
  DPF Canning + Umgebung1/1 -> Basis Berechnung1/6
  DPF Canning + Umgebung2/1 -> Basis Berechnung2/6
  DPF Canning + Umgebung3/1 -> Basis Berechnung3/6
  DPF Canning + Umgebung4/1 -> Basis Berechnung4/6
  DPF Canning + Umgebung5/1 -> Basis Berechnung5/6
  Mux4/1 -> Sum10/1, Demux1/1
  Mux5/1 -> Sum10/2, Demux2/1
  Mux6/1 -> Demux3/1, Sum10/3
  Mux7/1 -> Demux4/1, Sum10/4
  Mux8/1 -> Demux5/1, Sum10/5
  Mux9/1 -> Demux6/1, Sum10/6
  Gain3/1 -> DPF-Bel. alle Zonen/1  "m_Wasser_g"
  Subsystem/1(m_H2OAds_g) -> DPF-Bel. alle Zonen/4  "m_WasserAds_g"
  [KonfigParameters] -> Subsystem/2(Konfig), Subsystem1/2(Konfig)
  Mux14/1 -> DPF Zonentemp/1
  Subsystem1/1(m_H2OAds_g) -> Mux10/2, Sum6/2  "m_WasserAds_g"
  Sum6/1 -> [DPF_mWasserKond_g]
  Gain2/1 -> Sum6/1, Mux10/1  "m_Wasser_g"
  Mux10/1 -> DPF-Bel./1
  Sum13/1 -> Multiply/1
  Width/1 -> Multiply/2
  Multiply/1 -> DPF-Bel./4, Mux14/3  "T_DPF_avrg"
  Mux3/1 -> Sum13/1, Width/1, Mux14/1  "DPF Zonentemperatur"
  Konfig und TInit/1(Konfiguration) -> DPF Canning + Umgebung/3, DPF Canning + Umgebung1/3, DPF Canning + Umgebung2/3, DPF Canning + Umgebung3/3, DPF Canning + Umgebung4/3, DPF Canning + Umgebung5/3
  [T_Iso_Can_0] -> Mux16/1
  [T_Iso_Can_2] -> Mux16/3
  [T_Iso_Can_3] -> Mux16/4
  [T_Iso_Can_5] -> Mux16/6
  [T_Iso_Can_1] -> Mux16/2
  Mux16/1 -> DPF Iso-und-CanningTemp/1
  [T_Iso_Can_4] -> Mux16/5
  DPF Canning + Umgebung/2 -> [T_Iso_Can_0]
  DPF Canning + Umgebung1/2 -> [T_Iso_Can_1]
  DPF Canning + Umgebung2/2 -> [T_Iso_Can_2]
  DPF Canning + Umgebung3/2 -> [T_Iso_Can_3]
  DPF Canning + Umgebung4/2 -> [T_Iso_Can_4]
  DPF Canning + Umgebung5/2 -> [T_Iso_Can_5]
  Sum5/1 -> Sensordynamik Sensor 4/3, Druck nach DPF [mbar]/1
  Basis Berechnung5/3 -> Gain4/1, Massenstrom nach DPF [kg/s]/1
  Gain4/1 -> Sensordynamik Sensor 4/2  "dm_kgph"
  Sensordynamik Sensor 4/1 -> TnDPF_sim_Sensor_degC/1, Mux14/4
  Basis Berechnung5/4 -> Basis Berechnung4/5, Sensordynamik Sensor 4/1, Gastemperatur nach DPF [°C]/1, Basis Berechnung5/5, DPF Canning + Umgebung5/1, Mux3/6
  Konfiguration/1(Konfiguration) -> [KonfigParameters], Sensordynamik Sensor 4/4, Basis Berechnung5/7, Basis Berechnung4/7, Basis Berechnung3/7, Basis Berechnung2/7, Basis Berechnung1/7, Basis Berechnung/7, Konfig und TInit/1(ReInitTemp), Bus Selector/1

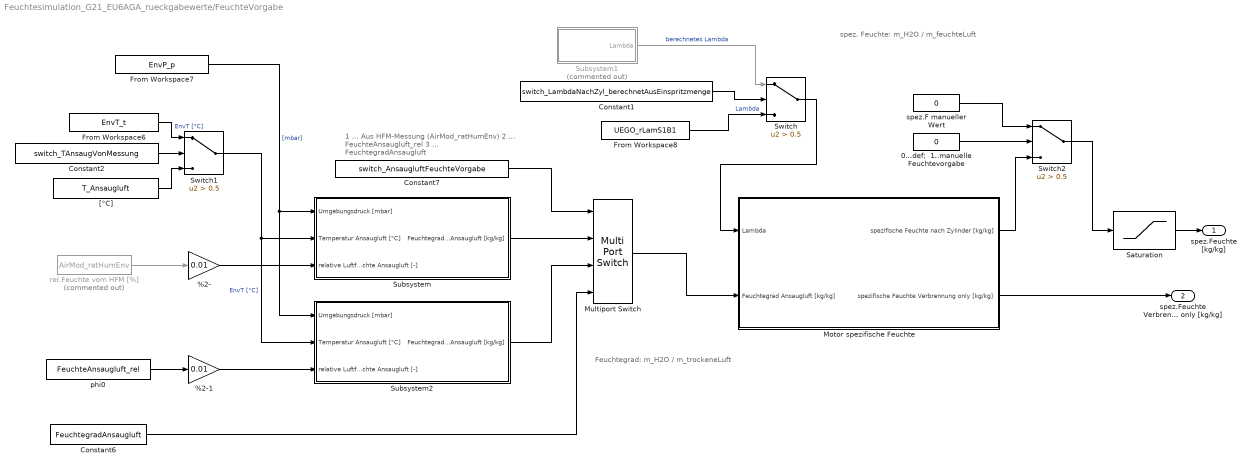
== system Feuchtesimulation_G21_EU6AGA_rueckgabewerte/FeuchteVorgabe ==
  note: 1 ... Aus HFM-Messung (AirMod_ratHumEnv)
      | 2 ... FeuchteAnsaugluft_rel
      | 3 ... FeuchtegradAnsaugluft
  note: Feuchtegrad: m_H2O / m_trockeneLuft
  note: spez. Feuchte: m_H2O / m_feuchteLuft
  %2- : Gain  Gain=0.01
  %2-1 : Gain  Gain=0.01
  0...def;  1..manuelle Feuchtevorgabe : Constant  Value=0
  Constant1 : Constant  Value=switch_LambdaNachZyl_berechnetAusEinspritzmenge
  Constant2 : Constant  Value=switch_TAnsaugVonMessung
  Constant6 : Constant  Value=FeuchtegradAnsaugluft
  Constant7 : Constant  Value=switch_AnsaugluftFeuchteVorgabe
  From Workspace6 : FromWorkspace  VariableName=EnvT_t  OutputAfterFinalValue=Holding final value
  From Workspace7 : FromWorkspace  VariableName=EnvP_p  OutputAfterFinalValue=Holding final value
  From Workspace8 : FromWorkspace  VariableName=UEGO_rLamS1B1  OutputAfterFinalValue=Holding final value
  Motor spezifische Feuchte : Subsystem
  Multiport Switch : MultiPortSwitch  DiagnosticForDefault=Warning
  Saturation : Saturate  UpperLimit=1  LowerLimit=0  RndMeth=Simplest
      settings: AttributesFormatString=Upper Limit = %<UpperLimit>\nLower Limit= %<LowerLimit>
  Subsystem : Subsystem
  Subsystem1 : Subsystem  Commented=on
  Subsystem2 : Subsystem
  Switch : Switch  Criteria=u2 > Threshold  Threshold=0.5
  Switch1 : Switch  Criteria=u2 > Threshold  Threshold=0.5
  Switch2 : Switch  Criteria=u2 > Threshold  Threshold=0.5
  "[°C]" : Constant  Value=T_Ansaugluft
  phi0 : Constant  Value=FeuchteAnsaugluft_rel
  rel.Feuchte vom HFM [%] : FromWorkspace  Commented=on  VariableName=AirMod_ratHumEnv
  spez.F manueller Wert : Constant  Value=0
  spez.Feuchte [kg/kg] : Outport  VectorParamsAs1DForOutWhenUnconnected=off
  spez.Feuchte Verbrennung only [kg/kg] : Outport  Port=2  VectorParamsAs1DForOutWhenUnconnected=off
  wires:
  Subsystem1/1(Lambda) -> Switch/1  "berechnetes Lambda"
  From Workspace7/1 -> Subsystem2/1(Umgebungsdruck [mbar]), Subsystem/1(Umgebungsdruck [mbar])  "[mbar]"
  %2-/1 -> Subsystem/3(relative Luftfeuchte Ansaugluft [-])
  Constant7/1 -> Multiport Switch/1
  Multiport Switch/1 -> Motor spezifische Feuchte/2(Feuchtegrad Ansaugluft [kg/kg])
  Constant6/1 -> Multiport Switch/4
  rel.Feuchte vom HFM [%]/1 -> %2-/1
  phi0/1 -> %2-1/1
  Switch1/1 -> Subsystem2/2(Temperatur Ansaugluft [°C]), Subsystem/2(Temperatur Ansaugluft [°C])  "EnvT [°C]"
  From Workspace8/1 -> Switch/3  "Lambda"
  %2-1/1 -> Subsystem2/3(relative Luftfeuchte Ansaugluft [-])
  Subsystem/1(Feuchtegrad Ansaugluft [kg/kg]) -> Multiport Switch/2
  Subsystem2/1(Feuchtegrad Ansaugluft [kg/kg]) -> Multiport Switch/3
  Constant1/1 -> Switch/2
  From Workspace6/1 -> Switch1/1  "EnvT [°C]"
  Constant2/1 -> Switch1/2
  "[°C]"/1 -> Switch1/3
  Motor spezifische Feuchte/2(spezifische Feuchte Verbrennung only [kg/kg]) -> spez.Feuchte Verbrennung only [kg/kg]/1
  Switch/1 -> Motor spezifische Feuchte/1(Lambda)
  0...def;  1..manuelle Feuchtevorgabe/1 -> Switch2/2
  spez.F manueller Wert/1 -> Switch2/1
  Saturation/1 -> spez.Feuchte [kg/kg]/1
  Motor spezifische Feuchte/1(spezifische Feuchte nach Zylinder [kg/kg]) -> Switch2/3
  Switch2/1 -> Saturation/1

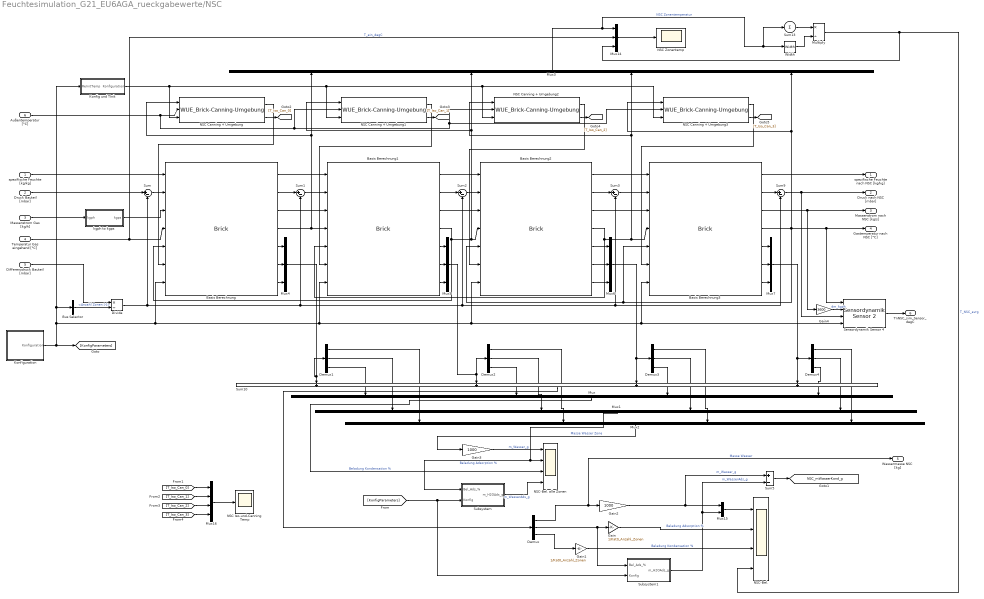
== system Feuchtesimulation_G21_EU6AGA_rueckgabewerte/NSC ==
  spezifische Feuchte [kg/kg] : Inport
  Druck Bauteil [mbar] : Inport  Port=2
  Massenstrom Gas [kg/h] : Inport  Port=3
  Temperatur Gas eingehend [°C] : Inport  Port=4
  Differenzdruck Bauteil [mbar] : Inport  Port=5
  Außentemperatur [°C] : Inport  Port=6
  Basis Berechnung{,1..3} (4 alike) : Feuchtesimulation_Lib/Brick  SystemSampleTime=-1  VariantActivationTime=update diagram  Latency=0  AutoFrameSizeCalculation=off
  Bus Selector : BusSelector  OutputSignals=Anzahl Zonen [-]
  Demux{,1..4} (5 alike) : Demux  Outputs=3
  Divide : Product  Inputs=*/
  Gain : Gain  Gain=1/Kat0_Anzahl_Zonen
  Gain1 : Gain  Gain=1/Kat0_Anzahl_Zonen
  Gain2 : Gain  Gain=1000
  Gain3 : Gain  Gain=1000
  Gain4 : Gain  Gain=3600
  Konfig und TInit : Subsystem
  Konfiguration : Subsystem
  Multiply : Product  Inputs=*/
  Mux{,1..3,16} (5 alike) : Mux
  Mux{4..7,14} (5 alike) : Mux  Inputs=3
  Mux15 : Mux  Inputs=2
  NSC Canning + Umgebung{,1..3} (4 alike) : Feuchtesimulation_Lib/WUE_Brick-Canning-Umgebung  SystemSampleTime=-1  VariantActivationTime=update diagram  Latency=0  AutoFrameSizeCalculation=off
  NSC Iso-und-CanningTemp : Scope
  NSC Zonentemp : Scope
  NSC-Bel. : Scope  NumInputPorts=4
  NSC-Bel. alle Zonen : Scope  NumInputPorts=4
  Sensordynamik Sensor 4 : Feuchtesimulation_Lib/Sensordynamik Sensor 2  SystemSampleTime=-1  VariantActivationTime=update diagram  Latency=0  AutoFrameSizeCalculation=off
  Subsystem : Subsystem
  Subsystem1 : Subsystem
  Sum{,1..3,9} (5 alike) : Sum  Inputs=|+-
  Sum10 : Sum  Inputs=++++
  Sum13 : Sum  Inputs=+
  Sum5 : Sum  Inputs=+-
  Width : Width
  kgph to kgps : Subsystem
  spezifische Feuchte nach NSC [kg/kg] : Outport  VectorParamsAs1DForOutWhenUnconnected=off
  Druck nach NSC [mbar] : Outport  Port=2  VectorParamsAs1DForOutWhenUnconnected=off
  Massenstrom nach NSC [kg/s] : Outport  Port=3  VectorParamsAs1DForOutWhenUnconnected=off
  Gastemperatur nach NSC [°C] : Outport  Port=4  VectorParamsAs1DForOutWhenUnconnected=off
  Wassermasse NSC [kg] : Outport  Port=5  VectorParamsAs1DForOutWhenUnconnected=off
  TnNSC_sim_Sensor_degC : Outport  Port=6  VectorParamsAs1DForOutWhenUnconnected=off
  tag scope: NSC_mWasserKond_g=global
  wires:
  Basis Berechnung3/6 -> Mux7/2
  Demux3/1 -> Mux2/3
  Demux1/1 -> Mux2/1
  Demux4/1 -> Mux2/4
  Demux2/1 -> Mux2/2
  Sum10/1 -> Demux/1
  Sum1/1 -> Basis Berechnung1/2
  Demux3/3 -> Mux/3
  Basis Berechnung3/5 -> Mux7/1
  Gain1/1 -> NSC-Bel./3  "Beladung Kondensation %"
  Temperatur Gas eingehend [°C]/1 -> Mux14/2, Basis Berechnung/4  "T_ein_degC"
  Demux/1 -> Wassermasse NSC [kg]/1, Gain2/1  "Masse Wasser"
  Basis Berechnung2/1 -> Basis Berechnung3/1
  Druck Bauteil [mbar]/1 -> Sum/1
  Basis Berechnung1/1 -> Basis Berechnung2/1
  spezifische Feuchte [kg/kg]/1 -> Basis Berechnung/1
  Basis Berechnung/4 -> Basis Berechnung1/4, NSC Canning + Umgebung/1, Mux3/1
  Basis Berechnung/1 -> Basis Berechnung1/1
  Mux1/1 -> NSC-Bel. alle Zonen/2, Subsystem/1(Bel_Ads_%)  "Beladung Adsorption %"
  Demux/3 -> Gain1/1
  Mux2/1 -> Gain3/1  "Masse Wasser Zone"
  Differenzdruck Bauteil [mbar]/1 -> Divide/1
  Sum2/1 -> Basis Berechnung2/2
  Demux4/3 -> Mux/4
  Demux1/2 -> Mux1/1
  Basis Berechnung2/2 -> Sum3/1
  Demux3/2 -> Mux1/3
  Basis Berechnung1/2 -> Sum2/1
  Demux1/3 -> Mux/1
  Mux3/1 -> Sum13/1, Width/1, Mux14/1  "NSC Zonentemperatur"
  Sum/1 -> Basis Berechnung/2
  Demux4/2 -> Mux1/4
  Mux/1 -> NSC-Bel. alle Zonen/3  "Beladung Kondensation %"
  Basis Berechnung/2 -> Sum1/1
  Basis Berechnung2/5 -> Mux6/1
  Demux2/3 -> Mux/2
  Demux2/2 -> Mux1/2
  Gain/1 -> NSC-Bel./2  "Beladung Adsorption %"
  Basis Berechnung3/4 -> Basis Berechnung3/5, Basis Berechnung2/5, NSC Canning + Umgebung3/1, Mux3/4, Sensordynamik Sensor 4/1, Gastemperatur nach NSC [°C]/1
  Massenstrom Gas [kg/h]/1 -> kgph to kgps/1(kgph)
  kgph to kgps/1(kgps) -> Basis Berechnung/3
  Basis Berechnung1/7 -> Mux5/3
  Basis Berechnung1/6 -> Mux5/2
  Basis Berechnung1/5 -> Mux5/1
  Basis Berechnung3/7 -> Mux7/3
  Basis Berechnung3/1 -> spezifische Feuchte nach NSC [kg/kg]/1
  Bus Selector/1 -> Divide/2  "<Anzahl Zonen [-]>"
  Basis Berechnung1/4 -> Basis Berechnung/5, Basis Berechnung2/4, NSC Canning + Umgebung1/1, Mux3/2
  Sum3/1 -> Basis Berechnung3/2
  Basis Berechnung2/6 -> Mux6/2
  Basis Berechnung2/3 -> Basis Berechnung3/3
  Basis Berechnung2/7 -> Mux6/3
  Basis Berechnung/3 -> Basis Berechnung1/3
  Sum9/1 -> Sensordynamik Sensor 4/3, Druck nach NSC [mbar]/1
  Basis Berechnung3/2 -> Sum9/1
  Basis Berechnung3/3 -> Gain4/1, Massenstrom nach NSC [kg/s]/1
  Basis Berechnung1/3 -> Basis Berechnung2/3
  Demux/2 -> Subsystem1/1(Bel_Ads_%), Gain/1
  Basis Berechnung2/4 -> Basis Berechnung1/5, Basis Berechnung3/4, Mux3/3, NSC Canning + Umgebung2/1
  Konfiguration/1(Konfiguration) -> [KonfigParameters], Sensordynamik Sensor 4/4, Basis Berechnung3/7, Basis Berechnung2/7, Basis Berechnung1/7, Basis Berechnung/7, Konfig und TInit/1(ReInitTemp), Bus Selector/1
  Divide/1 -> Sum9/2, Sum3/2, Sum2/2, Sum1/2, Sum/2
  Außentemperatur [°C]/1 -> NSC Canning + Umgebung3/2, NSC Canning + Umgebung2/2, NSC Canning + Umgebung1/2, NSC Canning + Umgebung/2
  NSC Canning + Umgebung3/1 -> Basis Berechnung3/6
  NSC Canning + Umgebung/1 -> Basis Berechnung/6
  NSC Canning + Umgebung1/1 -> Basis Berechnung1/6
  NSC Canning + Umgebung2/1 -> Basis Berechnung2/6
  Gain2/1 -> Mux15/1, Sum5/1  "m_Wasser_g"
  Basis Berechnung/5 -> Mux4/1
  Basis Berechnung/6 -> Mux4/2
  Basis Berechnung/7 -> Mux4/3
  Mux4/1 -> Demux1/1, Sum10/1
  Mux5/1 -> Demux2/1, Sum10/2
  Mux6/1 -> Sum10/3, Demux3/1
  Mux7/1 -> Sum10/4, Demux4/1
  Gain3/1 -> NSC-Bel. alle Zonen/1  "m_Wasser_g"
  [KonfigParameters] -> Subsystem/2(Konfig), Subsystem1/2(Konfig)
  Subsystem/1(m_H2OAds_g) -> NSC-Bel. alle Zonen/4  "m_WasserAds_g"
  Subsystem1/1(m_H2OAds_g) -> Sum5/2, Mux15/2  "m_WasserAds_g"
  Mux14/1 -> NSC Zonentemp/1
  Sum5/1 -> [NSC_mWasserKond_g]
  Mux15/1 -> NSC-Bel./1
  Sum13/1 -> Multiply/1
  Width/1 -> Multiply/2
  Multiply/1 -> NSC-Bel./4, Mux14/3  "T_NSC_avrg"
  Konfig und TInit/1(Konfiguration) -> NSC Canning + Umgebung3/3, NSC Canning + Umgebung2/3, NSC Canning + Umgebung1/3, NSC Canning + Umgebung/3
  NSC Canning + Umgebung/2 -> [T_Iso_Can_0]
  NSC Canning + Umgebung1/2 -> [T_Iso_Can_1]
  NSC Canning + Umgebung2/2 -> [T_Iso_Can_2]
  NSC Canning + Umgebung3/2 -> [T_Iso_Can_3]
  [T_Iso_Can_0] -> Mux16/1
  [T_Iso_Can_1] -> Mux16/2
  [T_Iso_Can_2] -> Mux16/3
  [T_Iso_Can_3] -> Mux16/4
  Mux16/1 -> NSC Iso-und-CanningTemp/1
  Gain4/1 -> Sensordynamik Sensor 4/2  "dm_kgph"
  Sensordynamik Sensor 4/1 -> TnNSC_sim_Sensor_degC/1

== system Feuchtesimulation_G21_EU6AGA_rueckgabewerte/Relative Feuchte [%] ==
  Spez F [kg/kg] : Inport
  Temp [°C] : Inport  Port=2
  Druck [mbar] : Inport  Port=3
  % : Gain  Gain=100
  1-D Lookup Table1 : Lookup_n-D  NumberOfTableDimensions=1  BreakpointsForDimension1=p_dsat.T  Table=p_dsat.p  ExtrapMethod=Clip  InternalRulePriority=Speed  RndMeth=Simplest  InputSameDT=on
  Divide : Product  Inputs=*/
  Limit Sättigungsdampfdruck : Subsystem
  Maximale spez Luftf.1 : MATLAB Function  TreatAsAtomicUnit=on
  Saturation2 : Saturate  UpperLimit=1  LowerLimit=0
  Rel F [%] : Outport  VectorParamsAs1DForOutWhenUnconnected=off
  wires:
  Spez F [kg/kg]/1 -> Divide/1
  Divide/1 -> %/1
  Temp [°C]/1 -> 1-D Lookup Table1/1
  Maximale spez Luftf.1/1(s_max) -> Saturation2/1
  Druck [mbar]/1 -> Limit Sättigungsdampfdruck/1(Druck [mbar]), Maximale spez Luftf.1/1(p)
  Saturation2/1 -> Divide/2
  1-D Lookup Table1/1 -> Limit Sättigungsdampfdruck/2(Sättigungsdampfdruck [mbar])
  Limit Sättigungsdampfdruck/1(Sättigungsdampfdruck Limitiert [mbar]) -> Maximale spez Luftf.1/2(p_dsat)
  %/1 -> Rel F [%]/1

== system Feuchtesimulation_G21_EU6AGA_rueckgabewerte/Relative Feuchte [%]1 ==
  Spez F [kg/kg] : Inport
  Temp [°C] : Inport  Port=2
  Druck [mbar] : Inport  Port=3
  % : Gain  Gain=100
  1-D Lookup Table1 : Lookup_n-D  NumberOfTableDimensions=1  BreakpointsForDimension1=p_dsat.T  Table=p_dsat.p  ExtrapMethod=Clip  InternalRulePriority=Speed  RndMeth=Simplest  InputSameDT=on
  <150% : Saturate  UpperLimit=150  LowerLimit=0
  Divide : Product  Inputs=*/
  Limit Sättigungsdampfdruck : Subsystem
  Maximale spez Luftf.1 : MATLAB Function  TreatAsAtomicUnit=on
  Saturation2 : Saturate  UpperLimit=1  LowerLimit=0
  Rel F [%] : Outport  VectorParamsAs1DForOutWhenUnconnected=off
  wires:
  Spez F [kg/kg]/1 -> Divide/1
  Divide/1 -> %/1
  Temp [°C]/1 -> 1-D Lookup Table1/1
  Maximale spez Luftf.1/1(s_max) -> Saturation2/1
  Druck [mbar]/1 -> Limit Sättigungsdampfdruck/1(Druck [mbar]), Maximale spez Luftf.1/1(p)
  Saturation2/1 -> Divide/2
  1-D Lookup Table1/1 -> Limit Sättigungsdampfdruck/2(Sättigungsdampfdruck [mbar])
  Limit Sättigungsdampfdruck/1(Sättigungsdampfdruck Limitiert [mbar]) -> Maximale spez Luftf.1/2(p_dsat)
  %/1 -> <150%/1
  <150%/1 -> Rel F [%]/1

== system Feuchtesimulation_G21_EU6AGA_rueckgabewerte/Relative Feuchte [%]2 ==
  Spez F [kg/kg] : Inport
  Temp [°C] : Inport  Port=2
  Druck [mbar] : Inport  Port=3
  % : Gain  Gain=100
  1-D Lookup Table1 : Lookup_n-D  NumberOfTableDimensions=1  BreakpointsForDimension1=p_dsat.T  Table=p_dsat.p  ExtrapMethod=Clip  InternalRulePriority=Speed  RndMeth=Simplest  InputSameDT=on
  Divide : Product  Inputs=*/
  Limit Sättigungsdampfdruck : Subsystem
  Maximale spez Luftf.1 : MATLAB Function  TreatAsAtomicUnit=on
  Saturation2 : Saturate  UpperLimit=1  LowerLimit=0
  Rel F [%] : Outport  VectorParamsAs1DForOutWhenUnconnected=off
  wires:
  Spez F [kg/kg]/1 -> Divide/1
  Divide/1 -> %/1
  Temp [°C]/1 -> 1-D Lookup Table1/1
  Maximale spez Luftf.1/1(s_max) -> Saturation2/1
  Druck [mbar]/1 -> Limit Sättigungsdampfdruck/1(Druck [mbar]), Maximale spez Luftf.1/1(p)
  Saturation2/1 -> Divide/2
  1-D Lookup Table1/1 -> Limit Sättigungsdampfdruck/2(Sättigungsdampfdruck [mbar])
  Limit Sättigungsdampfdruck/1(Sättigungsdampfdruck Limitiert [mbar]) -> Maximale spez Luftf.1/2(p_dsat)
  %/1 -> Rel F [%]/1

== system Feuchtesimulation_G21_EU6AGA_rueckgabewerte/Relative Feuchte [%]3 ==
  Spez F [kg/kg] : Inport
  Temp [°C] : Inport  Port=2
  Druck [mbar] : Inport  Port=3
  % : Gain  Gain=100
  1-D Lookup Table1 : Lookup_n-D  NumberOfTableDimensions=1  BreakpointsForDimension1=p_dsat.T  Table=p_dsat.p  ExtrapMethod=Clip  InternalRulePriority=Speed  RndMeth=Simplest  InputSameDT=on
  Divide : Product  Inputs=*/
  Limit Sättigungsdampfdruck : Subsystem
  Maximale spez Luftf.1 : MATLAB Function  TreatAsAtomicUnit=on
  Saturation2 : Saturate  UpperLimit=1  LowerLimit=0
  Rel F [%] : Outport  VectorParamsAs1DForOutWhenUnconnected=off
  wires:
  Spez F [kg/kg]/1 -> Divide/1
  Divide/1 -> %/1
  Temp [°C]/1 -> 1-D Lookup Table1/1
  Maximale spez Luftf.1/1(s_max) -> Saturation2/1
  Druck [mbar]/1 -> Limit Sättigungsdampfdruck/1(Druck [mbar]), Maximale spez Luftf.1/1(p)
  Saturation2/1 -> Divide/2
  1-D Lookup Table1/1 -> Limit Sättigungsdampfdruck/2(Sättigungsdampfdruck [mbar])
  Limit Sättigungsdampfdruck/1(Sättigungsdampfdruck Limitiert [mbar]) -> Maximale spez Luftf.1/2(p_dsat)
  %/1 -> Rel F [%]/1

== system Feuchtesimulation_G21_EU6AGA_rueckgabewerte/Relative Feuchte [%]4 ==
  Spez F [kg/kg] : Inport
  Temp [°C] : Inport  Port=2
  Druck [mbar] : Inport  Port=3
  % : Gain  Gain=100
  1-D Lookup Table1 : Lookup_n-D  NumberOfTableDimensions=1  BreakpointsForDimension1=p_dsat.T  Table=p_dsat.p  ExtrapMethod=Clip  InternalRulePriority=Speed  RndMeth=Simplest  InputSameDT=on
  Divide : Product  Inputs=*/
  Limit Sättigungsdampfdruck : Subsystem
  Maximale spez Luftf.1 : MATLAB Function  TreatAsAtomicUnit=on
  Saturation2 : Saturate  UpperLimit=1  LowerLimit=0
  Rel F [%] : Outport  VectorParamsAs1DForOutWhenUnconnected=off
  wires:
  Spez F [kg/kg]/1 -> Divide/1
  Divide/1 -> %/1
  Temp [°C]/1 -> 1-D Lookup Table1/1
  Maximale spez Luftf.1/1(s_max) -> Saturation2/1
  Druck [mbar]/1 -> Limit Sättigungsdampfdruck/1(Druck [mbar]), Maximale spez Luftf.1/1(p)
  Saturation2/1 -> Divide/2
  1-D Lookup Table1/1 -> Limit Sättigungsdampfdruck/2(Sättigungsdampfdruck [mbar])
  Limit Sättigungsdampfdruck/1(Sättigungsdampfdruck Limitiert [mbar]) -> Maximale spez Luftf.1/2(p_dsat)
  %/1 -> Rel F [%]/1

== system Feuchtesimulation_G21_EU6AGA_rueckgabewerte/Relative Feuchte [%]5 ==
  Spez F [kg/kg] : Inport
  Temp [°C] : Inport  Port=2
  Druck [mbar] : Inport  Port=3
  % : Gain  Gain=100
  1-D Lookup Table1 : Lookup_n-D  NumberOfTableDimensions=1  BreakpointsForDimension1=p_dsat.T  Table=p_dsat.p  ExtrapMethod=Clip  InternalRulePriority=Speed  RndMeth=Simplest  InputSameDT=on
  Divide : Product  Inputs=*/
  Limit Sättigungsdampfdruck : Subsystem
  Maximale spez Luftf.1 : MATLAB Function  TreatAsAtomicUnit=on
  Saturation2 : Saturate  UpperLimit=1  LowerLimit=0
  Rel F [%] : Outport  VectorParamsAs1DForOutWhenUnconnected=off
  wires:
  Spez F [kg/kg]/1 -> Divide/1
  Divide/1 -> %/1
  Temp [°C]/1 -> 1-D Lookup Table1/1
  Maximale spez Luftf.1/1(s_max) -> Saturation2/1
  Druck [mbar]/1 -> Limit Sättigungsdampfdruck/1(Druck [mbar]), Maximale spez Luftf.1/1(p)
  Saturation2/1 -> Divide/2
  1-D Lookup Table1/1 -> Limit Sättigungsdampfdruck/2(Sättigungsdampfdruck [mbar])
  Limit Sättigungsdampfdruck/1(Sättigungsdampfdruck Limitiert [mbar]) -> Maximale spez Luftf.1/2(p_dsat)
  %/1 -> Rel F [%]/1

== system Feuchtesimulation_G21_EU6AGA_rueckgabewerte/Relative Feuchte [%]6 ==
  Spez F [kg/kg] : Inport
  Temp [°C] : Inport  Port=2
  Druck [mbar] : Inport  Port=3
  % : Gain  Gain=100
  1-D Lookup Table1 : Lookup_n-D  NumberOfTableDimensions=1  BreakpointsForDimension1=p_dsat.T  Table=p_dsat.p  ExtrapMethod=Clip  InternalRulePriority=Speed  RndMeth=Simplest  InputSameDT=on
  Divide : Product  Inputs=*/
  Limit Sättigungsdampfdruck : Subsystem
  Maximale spez Luftf.1 : MATLAB Function  TreatAsAtomicUnit=on
  Saturation2 : Saturate  UpperLimit=1  LowerLimit=0
  Rel F [%] : Outport  VectorParamsAs1DForOutWhenUnconnected=off
  wires:
  Spez F [kg/kg]/1 -> Divide/1
  Divide/1 -> %/1
  Temp [°C]/1 -> 1-D Lookup Table1/1
  Maximale spez Luftf.1/1(s_max) -> Saturation2/1
  Druck [mbar]/1 -> Limit Sättigungsdampfdruck/1(Druck [mbar]), Maximale spez Luftf.1/1(p)
  Saturation2/1 -> Divide/2
  1-D Lookup Table1/1 -> Limit Sättigungsdampfdruck/2(Sättigungsdampfdruck [mbar])
  Limit Sättigungsdampfdruck/1(Sättigungsdampfdruck Limitiert [mbar]) -> Maximale spez Luftf.1/2(p_dsat)
  %/1 -> Rel F [%]/1
